simulink model "backlash_nonlinearity"  (R2024a)
settings: Solver=FixedStepAuto  StartTime=0.0  StopTime=40  FixedStep=1e-3  RelTol=1e-3
settings Model: Creator=Lenovo  LastModifiedBy=Lenovo

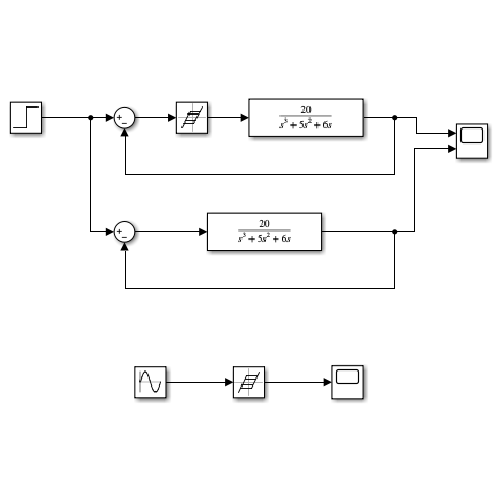
[thumbnail: Simulink's stored preview of the top-level diagram]
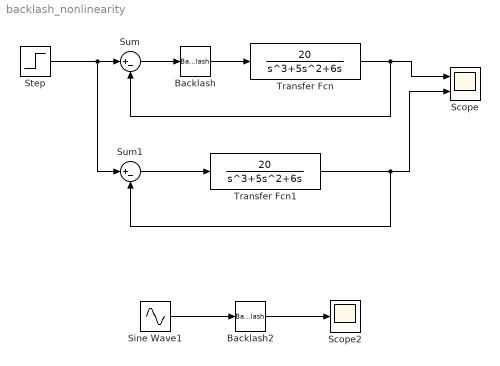
== system backlash_nonlinearity ==
  Backlash : Backlash  BacklashWidth=1.6
  Backlash2 : Backlash  BacklashWidth=1.6
  Scope : Scope  NumInputPorts=2
  Scope2 : Scope
  Sine Wave1 : Sin  SampleTime=0
  Step : Step  SampleTime=0
  Sum : Sum  Inputs=|+-
  Sum1 : Sum  Inputs=|+-
  Transfer Fcn : TransferFcn  Numerator=[20]  Denominator=[1 5 6 0]
  Transfer Fcn1 : TransferFcn  Numerator=[20]  Denominator=[1 5 6 0]
  wires:
  Step/1 -> Sum1/1, Sum/1
  Sum/1 -> Backlash/1
  Backlash/1 -> Transfer Fcn/1
  Transfer Fcn/1 -> Sum/2, Scope/1
  Sine Wave1/1 -> Backlash2/1
  Backlash2/1 -> Scope2/1
  Transfer Fcn1/1 -> Sum1/2, Scope/2
  Sum1/1 -> Transfer Fcn1/1
